simulink model "mdl_quadrotor_16b_Kopie"  (R2016b)
settings: Solver=ode4  StartTime=0.0  StopTime=20  FixedStep=0.0001  RelTol=1e-3
undefined symbols (not defined in the file or in its folder): Acc_uDot_mPerScnd2, Acc_vDot_mPerScnd2, Acc_wDot_mPerScnd2, Ag_phi_rad, Ag_psi_rad, Ag_theta_rad, AgVel_p_radPerScnd, AgVel_q_radPerScnd, AgVel_r_radPerScnd, par_mdlQuad, par_mdlQuadLin, Pos_x_mtr, Pos_y_mtr, Pos_z_mtr, V_u_mtrPerScnd, V_v_mtrPerScnd, V_w_mtrPerScnd
libraries: slident x4, vrlib x1
settings Model: Creator=Nu  LastModifiedBy=Nu

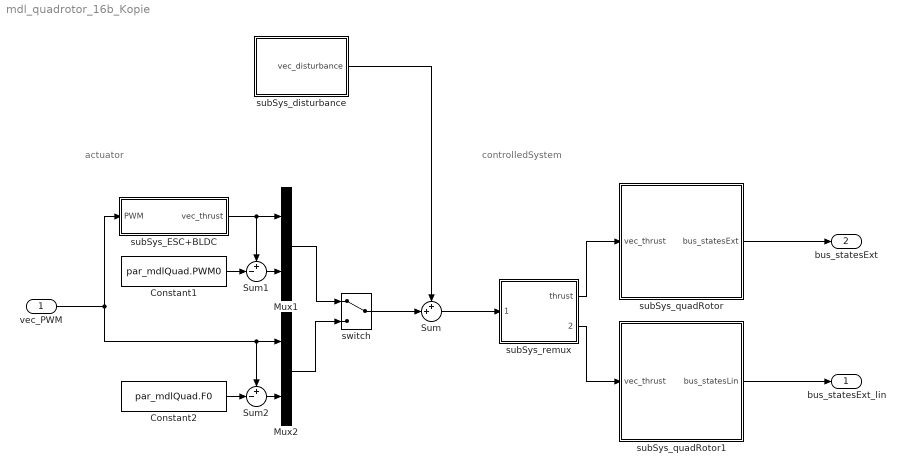
== system mdl_quadrotor_16b_Kopie ==
  note: controlledSystem
  note: actuator
  vec_PWM : Inport
  Constant1 : Constant  Value=par_mdlQuad.PWM0
  Constant2 : Constant  Value=par_mdlQuad.F0
  Mux1 : Mux  Inputs=2
  Mux2 : Mux  Inputs=2
  Sum : Sum  Inputs=++|
  Sum1 : Sum  Inputs=+-|
  Sum2 : Sum  Inputs=+-|
  subSys_ESC+BLDC : Subsystem
  subSys_disturbance : Subsystem
  subSys_quadRotor : Subsystem
  subSys_quadRotor1 : Subsystem
  subSys_remux : Subsystem
  switch : ManualSwitch
  bus_statesExt_lin : Outport  OutDataTypeStr=Bus: mdl_statesExt
  "bus_statesExt " : Outport  Port=2  OutDataTypeStr=Bus: mdl_statesExt
  wires:
  subSys_ESC+BLDC/1(vec_thrust) -> Sum1/1, Mux1/1
  subSys_quadRotor/1(bus_statesExt) -> "bus_statesExt "/1
  vec_PWM/1 -> subSys_ESC+BLDC/1(PWM), Mux2/1, Sum2/1
  subSys_disturbance/1(vec_disturbance) -> Sum/1
  subSys_quadRotor1/1(bus_statesLin) -> bus_statesExt_lin/1
  Constant2/1 -> Sum2/2
  Constant1/1 -> Sum1/2
  Mux1/1 -> switch/1
  switch/1 -> Sum/2
  Sum1/1 -> Mux1/2
  Mux2/1 -> switch/2
  Sum2/1 -> Mux2/2
  Sum/1 -> subSys_remux/1(thrust_all)
  subSys_remux/1(thrust) -> subSys_quadRotor/1(vec_thrust)
  subSys_remux/2(thrust_lin) -> subSys_quadRotor1/1(vec_thrust)

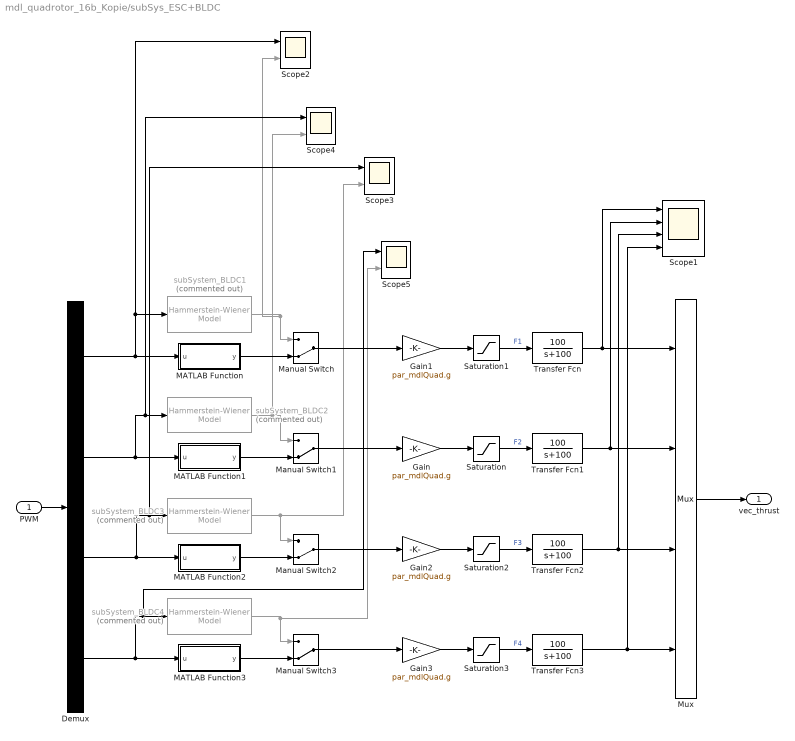
== system mdl_quadrotor_16b_Kopie/subSys_ESC+BLDC ==
  PWM : Inport
  Demux : Demux
  Gain{,1..3} (4 alike) : Gain  Gain=par_mdlQuad.g
  MATLAB Function : MATLAB Function  TreatAsAtomicUnit=on
  MATLAB Function1 : MATLAB Function  TreatAsAtomicUnit=on
  MATLAB Function2 : MATLAB Function  TreatAsAtomicUnit=on
  MATLAB Function3 : MATLAB Function  TreatAsAtomicUnit=on
  Manual Switch{,1..3} (4 alike) : ManualSwitch  CurrentSetting=0
  Mux : Mux
  Saturation{,1..3} (4 alike) : Saturate  UpperLimit=inf  LowerLimit=0
  Scope1 : Scope  NumInputPorts=4
  Scope{2..5} (4 alike) : Scope  NumInputPorts=2
  Transfer Fcn{,1..3} (4 alike) : TransferFcn  Numerator=[100]  Denominator=[1 100]
  subSystem_BLDC{1..4} (4 alike) : slident/Models/Hammerstein-Wiener Model  Commented=on  sys=nlhw1  IC=Zero  X0i=0
  vec_thrust : Outport
  wires:
  subSystem_BLDC1/1 -> Scope2/2, Manual Switch/1
  subSystem_BLDC2/1 -> Scope4/2, Manual Switch1/1
  subSystem_BLDC4/1 -> Scope5/2, Manual Switch3/1
  subSystem_BLDC3/1 -> Scope3/2, Manual Switch2/1
  Manual Switch/1 -> Gain1/1
  Manual Switch1/1 -> Gain/1
  Manual Switch2/1 -> Gain2/1
  Manual Switch3/1 -> Gain3/1
  Demux/2 -> Scope4/1, subSystem_BLDC2/1, MATLAB Function1/1(u)
  Demux/4 -> Scope5/1, subSystem_BLDC4/1, MATLAB Function3/1(u)
  Demux/1 -> Scope2/1, subSystem_BLDC1/1, MATLAB Function/1(u)
  Demux/3 -> Scope3/1, subSystem_BLDC3/1, MATLAB Function2/1(u)
  Saturation1/1 -> Transfer Fcn/1  "F1"
  Saturation/1 -> Transfer Fcn1/1  "F2"
  Saturation3/1 -> Transfer Fcn3/1  "F4"
  Saturation2/1 -> Transfer Fcn2/1  "F3"
  MATLAB Function/1(y) -> Manual Switch/2
  MATLAB Function1/1(y) -> Manual Switch1/2
  MATLAB Function2/1(y) -> Manual Switch2/2
  MATLAB Function3/1(y) -> Manual Switch3/2
  Gain1/1 -> Saturation1/1
  Gain/1 -> Saturation/1
  Gain2/1 -> Saturation2/1
  Gain3/1 -> Saturation3/1
  PWM/1 -> Demux/1
  Mux/1 -> vec_thrust/1
  Transfer Fcn/1 -> Scope1/1, Mux/1
  Transfer Fcn1/1 -> Scope1/2, Mux/2
  Transfer Fcn2/1 -> Scope1/3, Mux/3
  Transfer Fcn3/1 -> Scope1/4, Mux/4

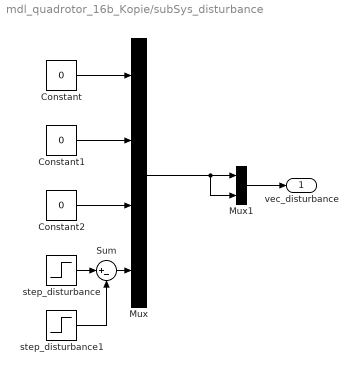
== system mdl_quadrotor_16b_Kopie/subSys_disturbance ==
  Constant : Constant  Value=0
  Constant1 : Constant  Value=0
  Constant2 : Constant  Value=0
  Mux : Mux
  Mux1 : Mux  Inputs=2
  Sum : Sum  Inputs=|+-
  step_disturbance : Step  Time=10  After=0.1  SampleTime=0
  step_disturbance1 : Step  Time=10.5  After=0.1  SampleTime=0
  vec_disturbance : Outport
  wires:
  Sum/1 -> Mux/4
  Constant/1 -> Mux/1
  Constant1/1 -> Mux/2
  Constant2/1 -> Mux/3
  Mux/1 -> Mux1/2, Mux1/1
  step_disturbance1/1 -> Sum/2
  step_disturbance/1 -> Sum/1
  Mux1/1 -> vec_disturbance/1

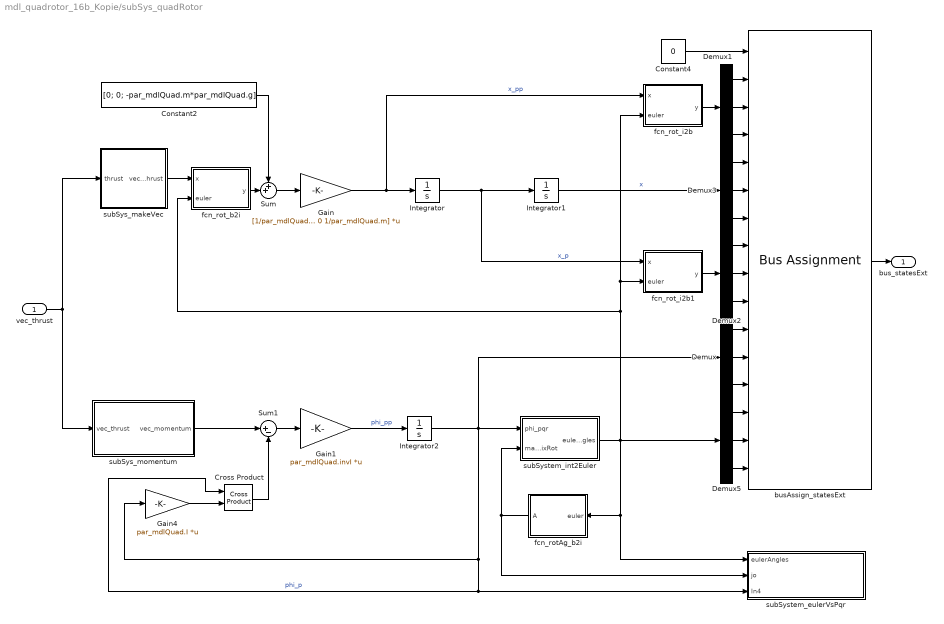
== system mdl_quadrotor_16b_Kopie/subSys_quadRotor ==
  vec_thrust : Inport
  Constant2 : Constant  Value=[0; 0; -par_mdlQuad.m*par_mdlQuad.g]
  Constant4 : Constant  Value=0  OutDataTypeStr=Bus: mdl_statesExt
  Cross Product : vrlib/Utilities/Cross Product
  Demux{,1..3,5} (5 alike) : Demux  Outputs=3
  Gain : Gain  Gain=[1/par_mdlQuad.m 0 0; 0 1/par_mdlQuad.m 0; 0 0 1/par_mdlQuad.m]  Multiplication=Matrix(K*u)
  Gain1 : Gain  Gain=par_mdlQuad.invI  Multiplication=Matrix(K*u)
  Gain4 : Gain  Gain=par_mdlQuad.I  Multiplication=Matrix(K*u)
  Integrator : Integrator
  Integrator1 : Integrator
  Integrator2 : Integrator
  Sum : Sum  Inputs=++|
  Sum1 : Sum  Inputs=|+-
  busAssign_statesExt : BusAssignment  AssignedSignals=Acc_uDot_mPerScnd2,Acc_vDot_mPerScnd2,Acc_wDot_mPerScnd2,Pos_x_mtr,Pos_y_mtr,Pos_z_mtr,V_u_mtrPerScnd,V_v_mtrPerScnd,V_w_mtrPerScnd,AgVel_p_radPerScnd,AgVel_q_radPerScnd,AgVel_r_radPerScnd,Ag_phi_rad,Ag_theta_rad,Ag_psi_rad
  fcn_rotAg_b2i : MATLAB Function  TreatAsAtomicUnit=on
  fcn_rot_b2i : MATLAB Function  TreatAsAtomicUnit=on
  fcn_rot_i2b : MATLAB Function  TreatAsAtomicUnit=on
  fcn_rot_i2b1 : MATLAB Function  TreatAsAtomicUnit=on
  subSys_makeVec : Subsystem
  subSys_momentum : Subsystem
  subSystem_eulerVsPqr : Subsystem
  subSystem_int2Euler : Subsystem
  bus_statesExt : Outport
  wires:
  fcn_rotAg_b2i/1(A) -> subSystem_eulerVsPqr/2(jo), subSystem_int2Euler/2(matrixRot)
  Constant2/1 -> Sum/1
  Sum/1 -> Gain/1
  Gain/1 -> fcn_rot_i2b/1(x), Integrator/1  "x_pp"
  Integrator/1 -> fcn_rot_i2b1/1(x), Integrator1/1  "x_p"
  Integrator1/1 -> Demux3/1  "x"
  Integrator2/1 -> Cross Product/1, subSystem_eulerVsPqr/3(In4), Gain4/1, Demux/1, subSystem_int2Euler/1(phi_pqr)  "phi_p"
  Gain1/1 -> Integrator2/1  "phi_pp"
  Sum1/1 -> Gain1/1
  Gain4/1 -> Cross Product/2
  Cross Product/1 -> Sum1/2
  Demux1/1 -> busAssign_statesExt/2
  Demux1/2 -> busAssign_statesExt/3
  Demux1/3 -> busAssign_statesExt/4
  Demux2/1 -> busAssign_statesExt/8
  Demux2/2 -> busAssign_statesExt/9
  Demux2/3 -> busAssign_statesExt/10
  Constant4/1 -> busAssign_statesExt/1
  busAssign_statesExt/1 -> bus_statesExt/1
  Demux/2 -> busAssign_statesExt/12
  Demux/1 -> busAssign_statesExt/11
  Demux/3 -> busAssign_statesExt/13
  Demux3/1 -> busAssign_statesExt/5
  Demux3/2 -> busAssign_statesExt/6
  Demux3/3 -> busAssign_statesExt/7
  Demux5/2 -> busAssign_statesExt/15
  Demux5/1 -> busAssign_statesExt/14
  Demux5/3 -> busAssign_statesExt/16
  vec_thrust/1 -> subSys_momentum/1(vec_thrust), subSys_makeVec/1(thrust)
  subSys_momentum/1(vec_momentum) -> Sum1/1
  subSystem_int2Euler/1(eulerAngles) -> subSystem_eulerVsPqr/1(eulerAngles), fcn_rotAg_b2i/1(euler), Demux5/1, fcn_rot_b2i/2(euler), fcn_rot_i2b/2(euler), fcn_rot_i2b1/2(euler)
  subSys_makeVec/1(vec_thrust) -> fcn_rot_b2i/1(x)
  fcn_rot_i2b/1(y) -> Demux1/1
  fcn_rot_b2i/1(y) -> Sum/2
  fcn_rot_i2b1/1(y) -> Demux2/1

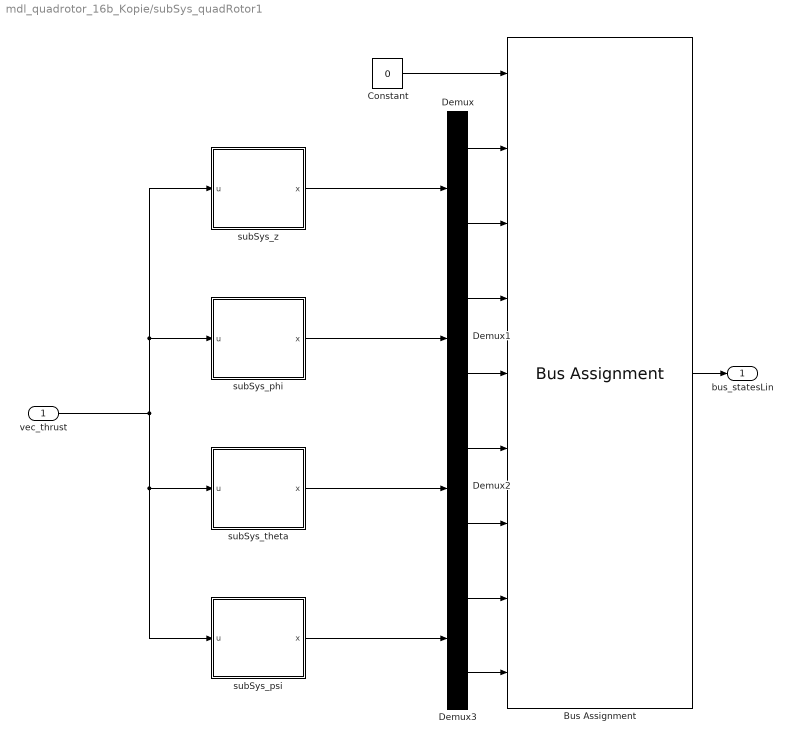
== system mdl_quadrotor_16b_Kopie/subSys_quadRotor1 ==
  vec_thrust : Inport
  Bus Assignment : BusAssignment  AssignedSignals=Pos_z_mtr,V_w_mtrPerScnd,Ag_phi_rad,AgVel_p_radPerScnd,Ag_theta_rad,AgVel_q_radPerScnd,Ag_psi_rad,AgVel_r_radPerScnd
  Constant : Constant  Value=0  OutDataTypeStr=Bus: mdl_statesExt
  Demux{,1..3} (4 alike) : Demux  Outputs=2
  subSys_phi : Subsystem
  subSys_psi : Subsystem
  subSys_theta : Subsystem
  subSys_z : Subsystem
  bus_statesLin : Outport
  wires:
  vec_thrust/1 -> subSys_psi/1(u), subSys_theta/1(u), subSys_phi/1(u), subSys_z/1(u)
  Bus Assignment/1 -> bus_statesLin/1
  Constant/1 -> Bus Assignment/1
  Demux/1 -> Bus Assignment/2
  Demux/2 -> Bus Assignment/3
  Demux1/1 -> Bus Assignment/4
  Demux1/2 -> Bus Assignment/5
  Demux2/1 -> Bus Assignment/6
  Demux2/2 -> Bus Assignment/7
  Demux3/1 -> Bus Assignment/8
  Demux3/2 -> Bus Assignment/9
  subSys_theta/1(x) -> Demux2/1
  subSys_psi/1(x) -> Demux3/1
  subSys_z/1(x) -> Demux/1
  subSys_phi/1(x) -> Demux1/1

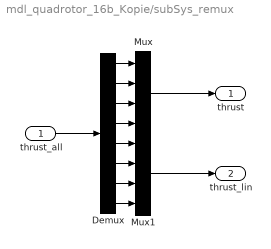
== system mdl_quadrotor_16b_Kopie/subSys_remux ==
  thrust_all : Inport
  Demux : Demux  Outputs=8
  Mux : Mux
  Mux1 : Mux
  thrust : Outport
  thrust_lin : Outport  Port=2
  wires:
  thrust_all/1 -> Demux/1
  Demux/1 -> Mux/1
  Demux/2 -> Mux/2
  Demux/3 -> Mux/3
  Demux/4 -> Mux/4
  Demux/5 -> Mux1/1
  Demux/6 -> Mux1/2
  Demux/7 -> Mux1/3
  Demux/8 -> Mux1/4
  Mux1/1 -> thrust_lin/1
  Mux/1 -> thrust/1

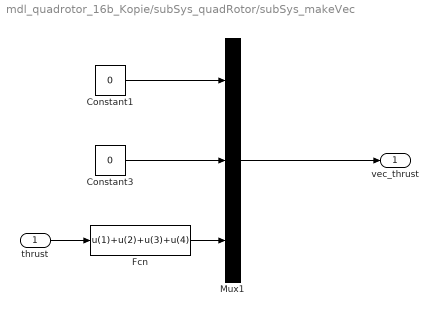
== system mdl_quadrotor_16b_Kopie/subSys_quadRotor/subSys_makeVec ==
  thrust : Inport
  Constant1 : Constant  Value=0
  Constant3 : Constant  Value=0
  Fcn : Fcn  Expr=u(1)+u(2)+u(3)+u(4)
  Mux1 : Mux  Inputs=3
  vec_thrust : Outport
  wires:
  Fcn/1 -> Mux1/3
  Constant1/1 -> Mux1/1
  Mux1/1 -> vec_thrust/1
  Constant3/1 -> Mux1/2
  thrust/1 -> Fcn/1

== system mdl_quadrotor_16b_Kopie/subSys_quadRotor/subSys_momentum ==
  vec_thrust : Inport
  Fcn : Fcn  Expr=(u(1)-u(3))*par_mdlQuad.l
  Fcn1 : Fcn  Expr=(u(2)-u(4))*par_mdlQuad.l
  Fcn2 : Fcn  Expr=(u(1)-u(3)+u(2)-u(4))*par_mdlQuad.gamma/par_mdlQuad.I(3,3)
  Mux : Mux  Inputs=3
  vec_momentum : Outport
  wires:
  Fcn/1 -> Mux/1
  Fcn1/1 -> Mux/2
  Fcn2/1 -> Mux/3
  Mux/1 -> vec_momentum/1
  vec_thrust/1 -> Fcn1/1, Fcn/1, Fcn2/1

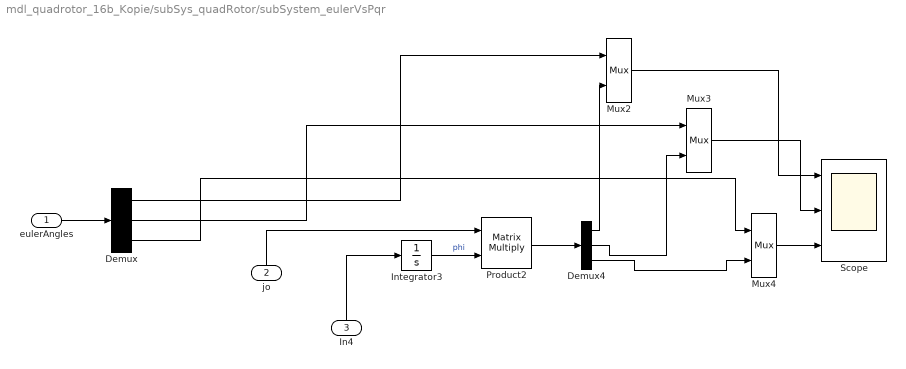
== system mdl_quadrotor_16b_Kopie/subSys_quadRotor/subSystem_eulerVsPqr ==
  eulerAngles : Inport
  jo : Inport  Port=2
  In4 : Inport  Port=3
  Demux : Demux  Outputs=3
  Demux4 : Demux  Outputs=3
  Integrator3 : Integrator
  Mux2 : Mux  Inputs=2
  Mux3 : Mux  Inputs=2
  Mux4 : Mux  Inputs=2
  Product2 : Product  Multiplication=Matrix(*)
  Scope : Scope  NumInputPorts=3
  wires:
  Integrator3/1 -> Product2/2  "phi"
  Mux2/1 -> Scope/1
  Product2/1 -> Demux4/1
  Demux4/1 -> Mux2/2
  Mux3/1 -> Scope/2
  Mux4/1 -> Scope/3
  Demux4/2 -> Mux3/2
  Demux4/3 -> Mux4/2
  In4/1 -> Integrator3/1
  jo/1 -> Product2/1
  eulerAngles/1 -> Demux/1
  Demux/1 -> Mux2/1
  Demux/2 -> Mux3/1
  Demux/3 -> Mux4/1

== system mdl_quadrotor_16b_Kopie/subSys_quadRotor/subSystem_int2Euler ==
  phi_pqr : Inport
  matrixRot : Inport  Port=2
  Integrator4 : Integrator
  Product1 : Product  Multiplication=Matrix(*)
  eulerAngles : Outport
  wires:
  Integrator4/1 -> eulerAngles/1
  Product1/1 -> Integrator4/1
  phi_pqr/1 -> Product1/2
  matrixRot/1 -> Product1/1

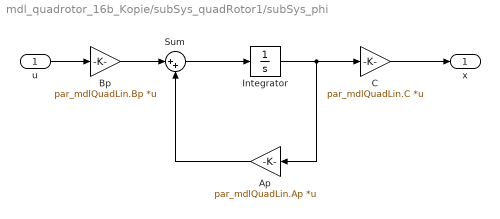
== system mdl_quadrotor_16b_Kopie/subSys_quadRotor1/subSys_phi ==
  u : Inport
  Ap : Gain  Gain=par_mdlQuadLin.Ap  Multiplication=Matrix(K*u)
  Bp : Gain  Gain=par_mdlQuadLin.Bp  Multiplication=Matrix(K*u)
  C : Gain  Gain=par_mdlQuadLin.C  Multiplication=Matrix(K*u)
  Integrator : Integrator
  Sum : Sum  Inputs=|++
  x : Outport
  wires:
  Ap/1 -> Sum/2
  C/1 -> x/1
  Integrator/1 -> C/1, Ap/1
  Sum/1 -> Integrator/1
  Bp/1 -> Sum/1
  u/1 -> Bp/1

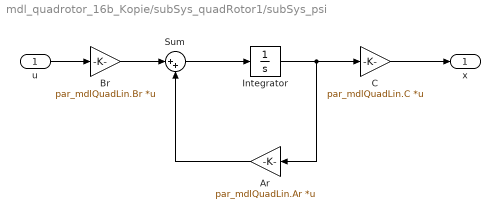
== system mdl_quadrotor_16b_Kopie/subSys_quadRotor1/subSys_psi ==
  u : Inport
  Ar : Gain  Gain=par_mdlQuadLin.Ar  Multiplication=Matrix(K*u)
  Br : Gain  Gain=par_mdlQuadLin.Br  Multiplication=Matrix(K*u)
  C : Gain  Gain=par_mdlQuadLin.C  Multiplication=Matrix(K*u)
  Integrator : Integrator
  Sum : Sum  Inputs=|++
  x : Outport
  wires:
  Ar/1 -> Sum/2
  C/1 -> x/1
  Integrator/1 -> C/1, Ar/1
  Sum/1 -> Integrator/1
  Br/1 -> Sum/1
  u/1 -> Br/1

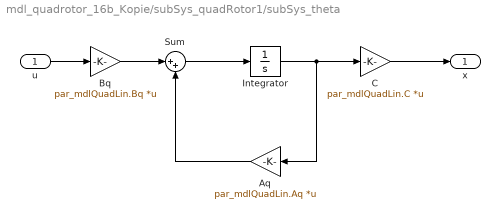
== system mdl_quadrotor_16b_Kopie/subSys_quadRotor1/subSys_theta ==
  u : Inport
  Aq : Gain  Gain=par_mdlQuadLin.Aq  Multiplication=Matrix(K*u)
  Bq : Gain  Gain=par_mdlQuadLin.Bq  Multiplication=Matrix(K*u)
  C : Gain  Gain=par_mdlQuadLin.C  Multiplication=Matrix(K*u)
  Integrator : Integrator
  Sum : Sum  Inputs=|++
  x : Outport
  wires:
  u/1 -> Bq/1
  Bq/1 -> Sum/1
  Sum/1 -> Integrator/1
  Integrator/1 -> Aq/1, C/1
  C/1 -> x/1
  Aq/1 -> Sum/2

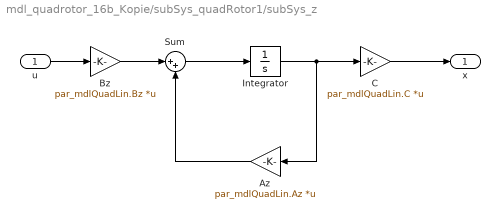
== system mdl_quadrotor_16b_Kopie/subSys_quadRotor1/subSys_z ==
  u : Inport
  Az : Gain  Gain=par_mdlQuadLin.Az  Multiplication=Matrix(K*u)
  Bz : Gain  Gain=par_mdlQuadLin.Bz  Multiplication=Matrix(K*u)
  C : Gain  Gain=par_mdlQuadLin.C  Multiplication=Matrix(K*u)
  Integrator : Integrator
  Sum : Sum  Inputs=|++
  x : Outport
  wires:
  u/1 -> Bz/1
  Bz/1 -> Sum/1
  Sum/1 -> Integrator/1
  Integrator/1 -> Az/1, C/1
  C/1 -> x/1
  Az/1 -> Sum/2

== matlab function mdl_quadrotor_16b_Kopie/subSys_quadRotor/fcn_rot_b2i ==
  data: x input; euler input; y output
function y = fcn(x, euler)

phi     = euler(1);
theta   = euler(2);
psi     = euler(3);

A       = mdl_rotEuler_zyx_b2i(phi, theta, psi);
y       = A*x;

== matlab function mdl_quadrotor_16b_Kopie/subSys_quadRotor/fcn_rot_i2b1 ==
  data: x input; euler input; y output
function y = fcn(x, euler)

phi     = euler(1);
theta   = euler(2);
psi     = euler(3);

A       = mdl_rotEuler_zyx_i2b(phi, theta, psi);
y       = A*x;

== matlab function mdl_quadrotor_16b_Kopie/subSys_ESC+BLDC/MATLAB Function ==
  data: u input; y output; par_mdlQuad parameter
function y = fcn(u, par_mdlQuad)

y = polyval(par_mdlQuad.coeffs, (u-par_mdlQuad.mean)/par_mdlQuad.std);

== matlab function mdl_quadrotor_16b_Kopie/subSys_ESC+BLDC/MATLAB Function1 ==
  data: u input; y output; par_mdlQuad parameter
function y = fcn(u, par_mdlQuad)

y = polyval(par_mdlQuad.coeffs, (u-par_mdlQuad.mean)/par_mdlQuad.std);

== matlab function mdl_quadrotor_16b_Kopie/subSys_ESC+BLDC/MATLAB Function2 ==
  data: u input; y output; par_mdlQuad parameter
function y = fcn(u, par_mdlQuad)

y = polyval(par_mdlQuad.coeffs, (u-par_mdlQuad.mean)/par_mdlQuad.std);

== matlab function mdl_quadrotor_16b_Kopie/subSys_ESC+BLDC/MATLAB Function3 ==
  data: u input; y output; par_mdlQuad parameter
function y = fcn(u, par_mdlQuad)

y = polyval(par_mdlQuad.coeffs, (u-par_mdlQuad.mean)/par_mdlQuad.std);

== matlab function mdl_quadrotor_16b_Kopie/subSys_quadRotor/fcn_rotAg_b2i ==
  data: euler input; A output
function A = fcn(euler)

phi     = euler(1);
theta   = euler(2);
psi     = euler(3);

A       = mdl_rotKarman_zyx_b2i(phi, theta, psi);

== matlab function mdl_quadrotor_16b_Kopie/subSys_quadRotor/fcn_rot_i2b ==
  data: x input; euler input; y output
function y = fcn(x, euler)

phi     = euler(1);
theta   = euler(2);
psi     = euler(3);

A       = mdl_rotEuler_zyx_i2b(phi, theta, psi);
y       = A*x;
